simulink model "Concave_hipp"  (R2023a)
settings: Solver=ode3  StartTime=0.0  StopTime=50  FixedStep=0.0001  RelTol=1e-3
values from neighbouring files (symbols this model uses):
  A = A1+A2    [dpdx_linearhipp.m]    (also in main_linear_hipp.m)
  B = [zeros(3,3);diag([1/M1,1/M2,1/M3])]    [dpdx_linearhipp.m]    (also in main_linear_hipp.m)
  Kall = cat(1,Kall,K_)    [main_linear_hipp.m]
  m = 3    [dpdx_linearhipp.m]    (also in main_linear_hipp.m = size(B',1))
  Pall = cat(1,Pall,P_)    [main_linear_hipp.m]
  R0q = Rb    [main_linear_hipp.m]
  rho = zeros(N,1)    [main_linear_hipp.m]
  rhospan = linspace(0,rhom,1000)    [main_linear_hipp.m]
  umax = [0.0288 0.5772 0.5772]    [main_linear_hipp.m]
  x0 = [pi/6;pi/4;pi/3;1;1;1]    [main_linear_hipp.m]
undefined symbols (not defined in the file or in its folder): Kb, Pb, Pcq
settings Model: Creator=fansh  LastModifiedBy=fansh
settings DebuggingCC: MultiTaskCondExecSysMsg=none  MultiTaskRateTransMsg=warning  TasksWithSamePriorityMsg=none  SigSpecEnsureSampleTimeMsg=none  UnknownTsInhSupMsg=none  SFUnexpectedBacktrackingDiag=none

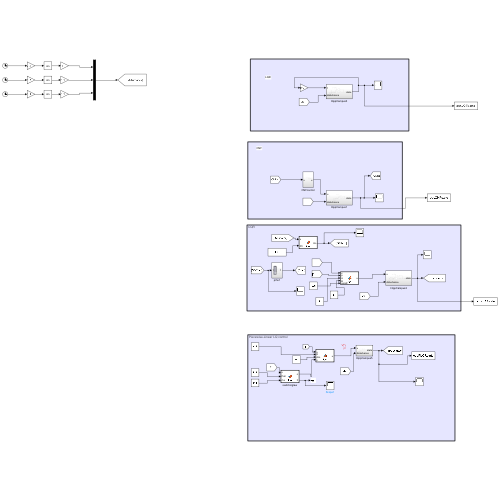
[thumbnail: Simulink's stored preview of the top-level diagram]
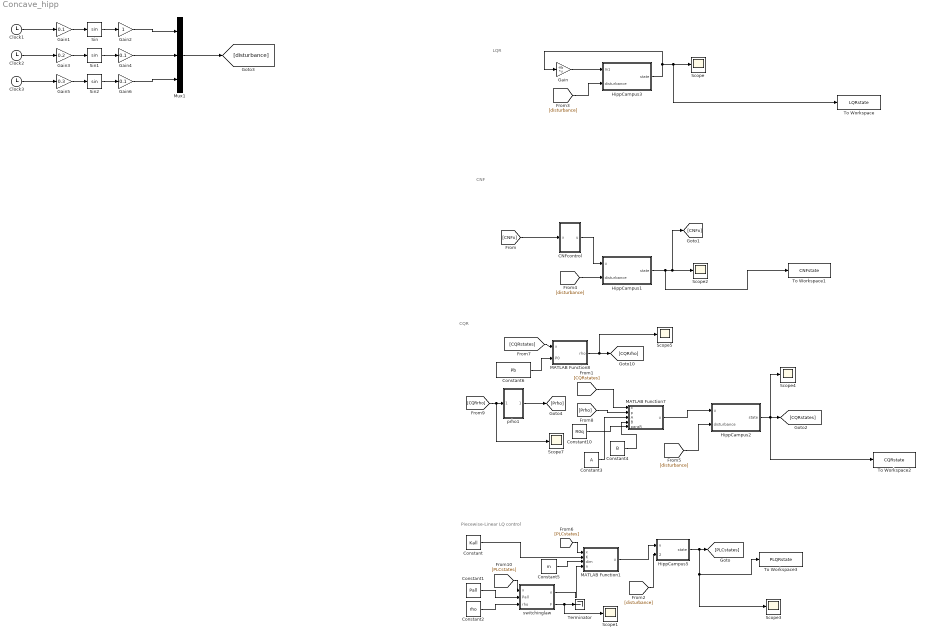
== system Concave_hipp ==
  note: CNF
  note: LQR
  note: CQR
  note: Piecewise-Linear LQ control
  CNFcontrol : Subsystem
  Clock1 : Clock
  Clock2 : Clock
  Clock3 : Clock
  Constant : Constant  Value=Kall
  Constant1 : Constant  Value=Pall
  Constant10 : Constant  Value=R0q
  Constant2 : Constant  Value=rho
  Constant3 : Constant  Value=A
  Constant4 : Constant  Value=B
  Constant5 : Constant  Value=m
  Constant6 : Constant  Value=Pb
  Gain : Gain  Gain=-Kb  Multiplication=Matrix(K*u)
  Gain1 : Gain  Gain=0.1
  Gain2 : Gain
  Gain3 : Gain  Gain=0.2
  Gain4 : Gain  Gain=0.1
  Gain5 : Gain  Gain=0.3
  Gain6 : Gain  Gain=0.1
  HippCampus1 : Subsystem
  HippCampus2 : Subsystem
  HippCampus3 : Subsystem
  HippCampus5 : Subsystem
  MATLAB Function1 : MATLAB Function  TreatAsAtomicUnit=on
  MATLAB Function7 : MATLAB Function  TreatAsAtomicUnit=on
  MATLAB Function8 : MATLAB Function  TreatAsAtomicUnit=on
  Mux1 : Mux  Inputs=3
  Scope{,1..5,7} (7 alike) : Scope
  Sin : Trigonometry
  Sin1 : Trigonometry
  Sin2 : Trigonometry
  Terminator : Terminator
  To Workspace : ToWorkspace  VariableName=LQRstate  SaveFormat=Timeseries  SampleTime=-1
  To Workspace1 : ToWorkspace  VariableName=CNFstate  SaveFormat=Timeseries  SampleTime=-1
  To Workspace2 : ToWorkspace  VariableName=CQRstate  SaveFormat=Timeseries  SampleTime=-1
  To Workspace3 : ToWorkspace  VariableName=PLQRstate  SaveFormat=Timeseries  SampleTime=-1
  prho1 : Subsystem
  switchinglaw : MATLAB Function  TreatAsAtomicUnit=on
  wires:
  HippCampus3/1(state) -> To Workspace/1, Scope/1, Gain/1
  Gain/1 -> HippCampus3/1(In1)
  Clock1/1 -> Gain1/1
  Gain1/1 -> Sin/1
  Sin/1 -> Gain2/1
  Sin1/1 -> Gain4/1
  Clock2/1 -> Gain3/1
  Gain3/1 -> Sin1/1
  Sin2/1 -> Gain6/1
  Clock3/1 -> Gain5/1
  Gain5/1 -> Sin2/1
  Gain2/1 -> Mux1/1
  Gain4/1 -> Mux1/2
  Gain6/1 -> Mux1/3
  Mux1/1 -> [disturbance]
  HippCampus1/1(state) -> To Workspace1/1, Scope2/1, [CNFx]
  [Prho] -> MATLAB Function7/2(p)
  [CQRrho] -> Scope7/1, prho1/1(In1)
  HippCampus2/1(state) -> To Workspace2/1, Scope4/1, [CQRstates]
  prho1/1(Out1) -> [Prho]
  Constant10/1 -> MATLAB Function7/5(paraR)
  MATLAB Function8/1(rho) -> Scope5/1, [CQRrho]
  [CQRstates] -> MATLAB Function8/1(x)
  Constant6/1 -> MATLAB Function8/2(P0)
  MATLAB Function7/1(u) -> HippCampus2/1(u)
  [CQRstates] -> MATLAB Function7/1(x)
  [disturbance] -> HippCampus3/2(disturbance)
  [disturbance] -> HippCampus1/2(disturbance)
  [CNFx] -> CNFcontrol/1(x)
  CNFcontrol/1(u) -> HippCampus1/1(u)
  [disturbance] -> HippCampus2/2(disturbance)
  Constant/1 -> MATLAB Function1/2(K)
  [PLCstates] -> switchinglaw/1(x)
  switchinglaw/2(F) -> Scope1/1, Terminator/1
  switchinglaw/1(n) -> MATLAB Function1/4(n)
  HippCampus5/1(state) -> Scope3/1, To Workspace3/1, [PLCstates]
  ? -> ?
  [PLCstates] -> MATLAB Function1/1(x)
  Constant1/1 -> switchinglaw/2(Pall)
  MATLAB Function1/1(u) -> HippCampus5/1(u)
  Constant2/1 -> switchinglaw/3(rho)
  Constant5/1 -> MATLAB Function1/3(dim)
  [disturbance] -> HippCampus5/2(disturbance)
  Constant3/1 -> MATLAB Function7/3(A)
  Constant4/1 -> MATLAB Function7/4(B)

== system Concave_hipp/CNFcontrol ==
  x : Inport
  Constant : Constant  Value=200
  Constant1 : Constant  Value=Kb
  Constant2 : Constant  Value=Pb
  MATLAB Function1 : MATLAB Function  TreatAsAtomicUnit=on
  MATLAB Function2 : MATLAB Function  TreatAsAtomicUnit=on
  u : Outport
  wires:
  MATLAB Function2/1(rho) -> MATLAB Function1/3(rho)
  MATLAB Function1/1(u) -> u/1
  x/1 -> MATLAB Function2/1(x), MATLAB Function1/1(x)
  Constant/1 -> MATLAB Function1/4(k)
  Constant1/1 -> MATLAB Function1/2(Kb)
  Constant2/1 -> MATLAB Function2/2(Pb)

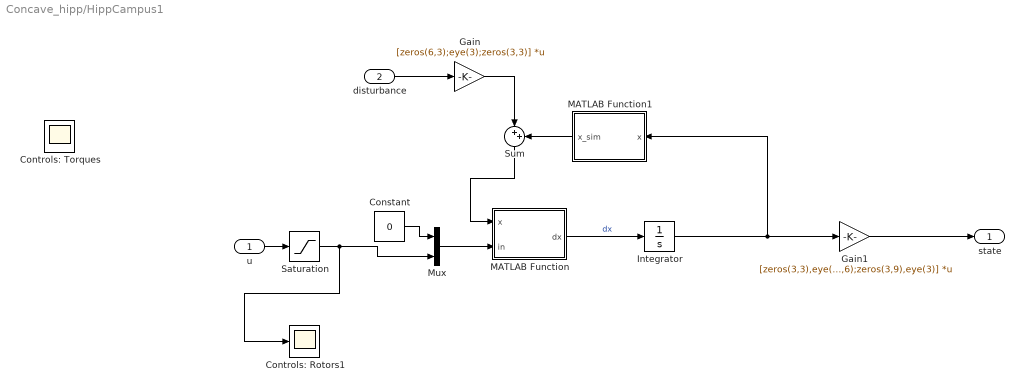
== system Concave_hipp/HippCampus1 ==
  u : Inport
  disturbance : Inport  Port=2
  Constant : Constant  Value=0
  Controls: Rotors1 : Scope
  Controls: Torques : Scope
  Gain : Gain  Gain=[zeros(6,3);eye(3);zeros(3,3)]  Multiplication=Matrix(K*u)
  Gain1 : Gain  Gain=[zeros(3,3),eye(3),zeros(3,6);zeros(3,9),eye(3)]  Multiplication=Matrix(K*u)
  Integrator : Integrator  InitialCondition=[zeros(3,1);x0(1:3);zeros(3,1);x0(4:6)]
  MATLAB Function : MATLAB Function  TreatAsAtomicUnit=on
  MATLAB Function1 : MATLAB Function  TreatAsAtomicUnit=on
  Mux : Mux  Inputs=2
  Saturation : Saturate  UpperLimit=umax'  LowerLimit=-umax'
  Sum : Sum  Inputs=|++
  state : Outport
  wires:
  MATLAB Function/1(dx) -> Integrator/1  "dx"
  Integrator/1 -> Gain1/1, MATLAB Function1/1(x)
  disturbance/1 -> Gain/1
  Gain/1 -> Sum/1
  Sum/1 -> MATLAB Function/1(x)
  MATLAB Function1/1(x_sim) -> Sum/2
  Gain1/1 -> state/1
  Mux/1 -> MATLAB Function/2(in)
  Saturation/1 -> Controls: Rotors1/1, Mux/2
  Constant/1 -> Mux/1
  u/1 -> Saturation/1

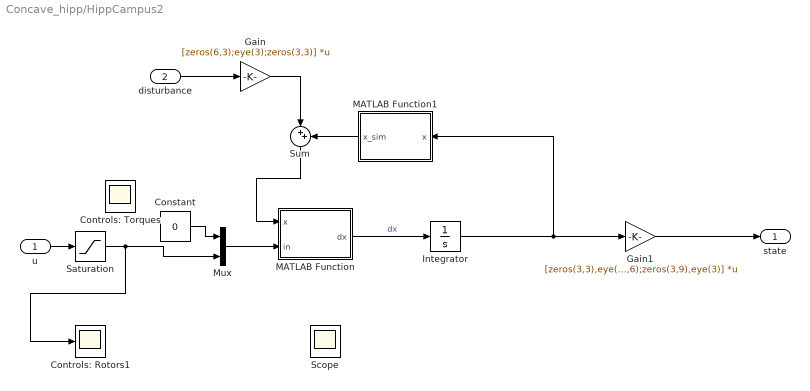
== system Concave_hipp/HippCampus2 ==
  u : Inport
  disturbance : Inport  Port=2
  Constant : Constant  Value=0
  Controls: Rotors1 : Scope
  Controls: Torques : Scope
  Gain : Gain  Gain=[zeros(6,3);eye(3);zeros(3,3)]  Multiplication=Matrix(K*u)
  Gain1 : Gain  Gain=[zeros(3,3),eye(3),zeros(3,6);zeros(3,9),eye(3)]  Multiplication=Matrix(K*u)
  Integrator : Integrator  InitialCondition=[zeros(3,1);x0(1:3);zeros(3,1);x0(4:6)]
  MATLAB Function : MATLAB Function  TreatAsAtomicUnit=on
  MATLAB Function1 : MATLAB Function  TreatAsAtomicUnit=on
  Mux : Mux  Inputs=2
  Saturation : Saturate  UpperLimit=umax'  LowerLimit=-umax'
  Scope : Scope
  Sum : Sum  Inputs=|++
  state : Outport
  wires:
  MATLAB Function/1(dx) -> Integrator/1  "dx"
  Integrator/1 -> Gain1/1, MATLAB Function1/1(x)
  disturbance/1 -> Gain/1
  Gain/1 -> Sum/1
  Sum/1 -> MATLAB Function/1(x)
  MATLAB Function1/1(x_sim) -> Sum/2
  Gain1/1 -> state/1
  Mux/1 -> MATLAB Function/2(in)
  Saturation/1 -> Controls: Rotors1/1, Mux/2
  Constant/1 -> Mux/1
  u/1 -> Saturation/1
  ? -> Scope/1

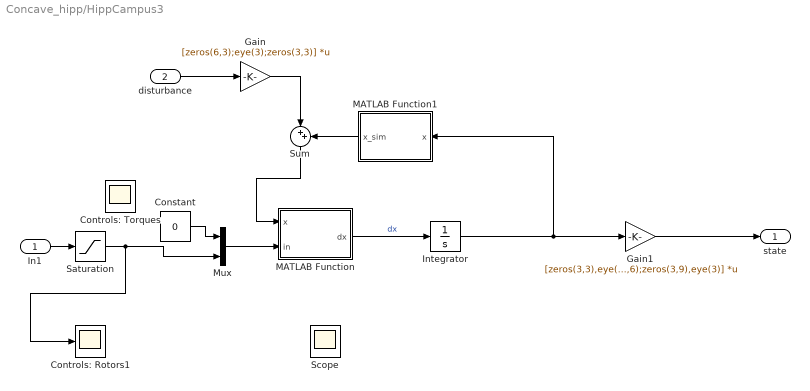
== system Concave_hipp/HippCampus3 ==
  In1 : Inport
  disturbance : Inport  Port=2
  Constant : Constant  Value=0
  Controls: Rotors1 : Scope
  Controls: Torques : Scope
  Gain : Gain  Gain=[zeros(6,3);eye(3);zeros(3,3)]  Multiplication=Matrix(K*u)
  Gain1 : Gain  Gain=[zeros(3,3),eye(3),zeros(3,6);zeros(3,9),eye(3)]  Multiplication=Matrix(K*u)
  Integrator : Integrator  InitialCondition=[zeros(3,1);x0(1:3);zeros(3,1);x0(4:6)]
  MATLAB Function : MATLAB Function  TreatAsAtomicUnit=on
  MATLAB Function1 : MATLAB Function  TreatAsAtomicUnit=on
  Mux : Mux  Inputs=2
  Saturation : Saturate  UpperLimit=umax'  LowerLimit=-umax'
  Scope : Scope
  Sum : Sum  Inputs=|++
  state : Outport
  wires:
  MATLAB Function/1(dx) -> Integrator/1  "dx"
  Integrator/1 -> Gain1/1, MATLAB Function1/1(x)
  disturbance/1 -> Gain/1
  Gain/1 -> Sum/1
  Sum/1 -> MATLAB Function/1(x)
  MATLAB Function1/1(x_sim) -> Sum/2
  Gain1/1 -> state/1
  Mux/1 -> MATLAB Function/2(in)
  Saturation/1 -> Controls: Rotors1/1, Mux/2
  Constant/1 -> Mux/1
  In1/1 -> Saturation/1
  ? -> Scope/1

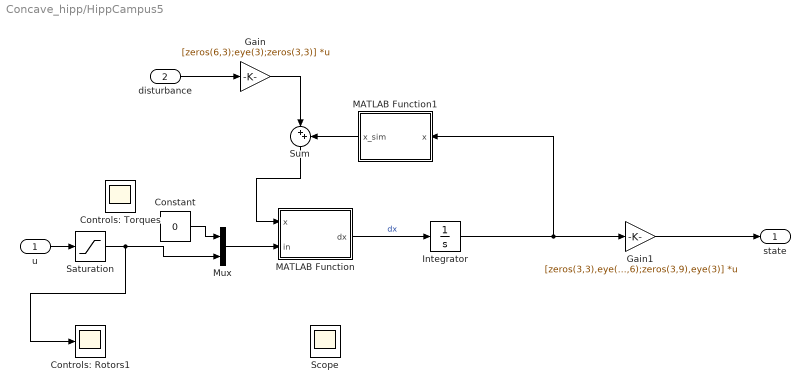
== system Concave_hipp/HippCampus5 ==
  u : Inport
  disturbance : Inport  Port=2
  Constant : Constant  Value=0
  Controls: Rotors1 : Scope
  Controls: Torques : Scope
  Gain : Gain  Gain=[zeros(6,3);eye(3);zeros(3,3)]  Multiplication=Matrix(K*u)
  Gain1 : Gain  Gain=[zeros(3,3),eye(3),zeros(3,6);zeros(3,9),eye(3)]  Multiplication=Matrix(K*u)
  Integrator : Integrator  InitialCondition=[zeros(3,1);x0(1:3);zeros(3,1);x0(4:6)]
  MATLAB Function : MATLAB Function  TreatAsAtomicUnit=on
  MATLAB Function1 : MATLAB Function  TreatAsAtomicUnit=on
  Mux : Mux  Inputs=2
  Saturation : Saturate  UpperLimit=umax'  LowerLimit=-umax'
  Scope : Scope
  Sum : Sum  Inputs=|++
  state : Outport
  wires:
  MATLAB Function/1(dx) -> Integrator/1  "dx"
  Integrator/1 -> Gain1/1, MATLAB Function1/1(x)
  disturbance/1 -> Gain/1
  Gain/1 -> Sum/1
  Sum/1 -> MATLAB Function/1(x)
  MATLAB Function1/1(x_sim) -> Sum/2
  Gain1/1 -> state/1
  Mux/1 -> MATLAB Function/2(in)
  Saturation/1 -> Controls: Rotors1/1, Mux/2
  Constant/1 -> Mux/1
  u/1 -> Saturation/1
  ? -> Scope/1

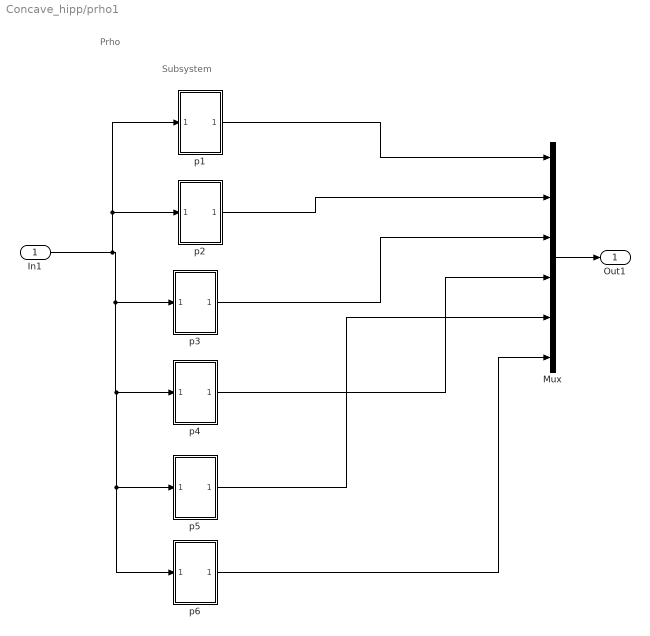
== system Concave_hipp/prho1 ==
  note: Prho
  note: Subsystem
  In1 : Inport
  Mux : Mux  Inputs=6
  p1 : Subsystem
  p2 : Subsystem
  p3 : Subsystem
  p4 : Subsystem
  p5 : Subsystem
  p6 : Subsystem
  Out1 : Outport
  wires:
  p4/1(Out1) -> Mux/4
  In1/1 -> p6/1(In1), p5/1(In1), p4/1(In1), p3/1(In1), p2/1(In1), p1/1(In1)
  Mux/1 -> Out1/1
  p1/1(Out1) -> Mux/1
  p3/1(Out1) -> Mux/3
  p2/1(Out1) -> Mux/2
  p5/1(Out1) -> Mux/5
  p6/1(Out1) -> Mux/6

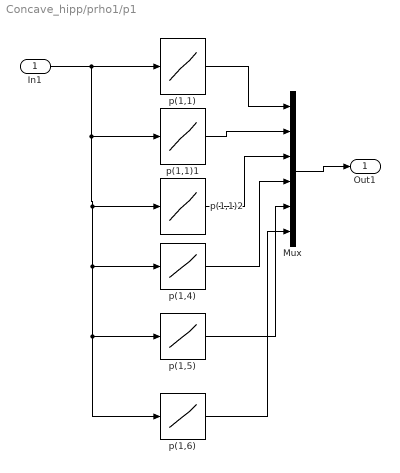
== system Concave_hipp/prho1/p1 ==
  In1 : Inport
  Mux : Mux  Inputs=6
  p(1,1) : Lookup_n-D  NumberOfTableDimensions=1  BreakpointsForDimension1=rhospan  Table=Pcq(:,1)  InterpMethod=Linear Lagrange  InternalRulePriority=Speed  RndMeth=Simplest
  p(1,1)1 : Lookup_n-D  NumberOfTableDimensions=1  BreakpointsForDimension1=rhospan  Table=Pcq(:,2)  InterpMethod=Linear Lagrange  InternalRulePriority=Speed  RndMeth=Simplest
  p(1,1)2 : Lookup_n-D  NumberOfTableDimensions=1  BreakpointsForDimension1=rhospan  Table=Pcq(:,3)  InterpMethod=Linear Lagrange  InternalRulePriority=Speed  RndMeth=Simplest
  p(1,4) : Lookup_n-D  NumberOfTableDimensions=1  BreakpointsForDimension1=rhospan  Table=Pcq(:,4)  InterpMethod=Linear Lagrange  InternalRulePriority=Speed  RndMeth=Simplest
  p(1,5) : Lookup_n-D  NumberOfTableDimensions=1  BreakpointsForDimension1=rhospan  Table=Pcq(:,5)  InterpMethod=Linear Lagrange  InternalRulePriority=Speed  RndMeth=Simplest
  p(1,6) : Lookup_n-D  NumberOfTableDimensions=1  BreakpointsForDimension1=rhospan  Table=Pcq(:,6)  InterpMethod=Linear Lagrange  InternalRulePriority=Speed  RndMeth=Simplest
  Out1 : Outport
  wires:
  p(1,1)1/1 -> Mux/2
  p(1,4)/1 -> Mux/4
  In1/1 -> p(1,1)1/1, p(1,1)2/1, p(1,6)/1, p(1,5)/1, p(1,4)/1, p(1,1)/1
  p(1,1)/1 -> Mux/1
  p(1,1)2/1 -> Mux/3
  Mux/1 -> Out1/1
  p(1,5)/1 -> Mux/5
  p(1,6)/1 -> Mux/6

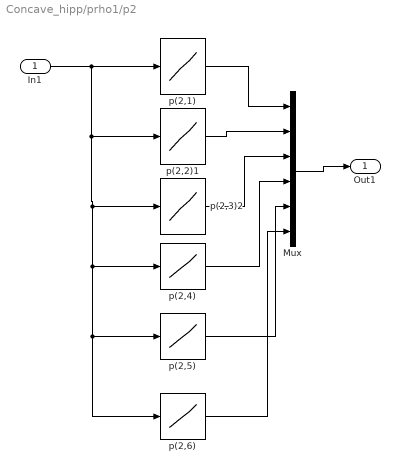
== system Concave_hipp/prho1/p2 ==
  In1 : Inport
  Mux : Mux  Inputs=6
  p(2,1) : Lookup_n-D  NumberOfTableDimensions=1  BreakpointsForDimension1=rhospan  Table=Pcq(:,7)  InterpMethod=Linear Lagrange  InternalRulePriority=Speed  RndMeth=Simplest
  p(2,2)1 : Lookup_n-D  NumberOfTableDimensions=1  BreakpointsForDimension1=rhospan  Table=Pcq(:,8)  InterpMethod=Linear Lagrange  InternalRulePriority=Speed  RndMeth=Simplest
  p(2,3)2 : Lookup_n-D  NumberOfTableDimensions=1  BreakpointsForDimension1=rhospan  Table=Pcq(:,9)  InterpMethod=Linear Lagrange  InternalRulePriority=Speed  RndMeth=Simplest
  p(2,4) : Lookup_n-D  NumberOfTableDimensions=1  BreakpointsForDimension1=rhospan  Table=Pcq(:,10)  InterpMethod=Linear Lagrange  InternalRulePriority=Speed  RndMeth=Simplest
  p(2,5) : Lookup_n-D  NumberOfTableDimensions=1  BreakpointsForDimension1=rhospan  Table=Pcq(:,11)  InterpMethod=Linear Lagrange  InternalRulePriority=Speed  RndMeth=Simplest
  p(2,6) : Lookup_n-D  NumberOfTableDimensions=1  BreakpointsForDimension1=rhospan  Table=Pcq(:,12)  InterpMethod=Linear Lagrange  InternalRulePriority=Speed  RndMeth=Simplest
  Out1 : Outport
  wires:
  p(2,2)1/1 -> Mux/2
  p(2,4)/1 -> Mux/4
  In1/1 -> p(2,2)1/1, p(2,3)2/1, p(2,6)/1, p(2,5)/1, p(2,4)/1, p(2,1)/1
  p(2,1)/1 -> Mux/1
  p(2,3)2/1 -> Mux/3
  Mux/1 -> Out1/1
  p(2,5)/1 -> Mux/5
  p(2,6)/1 -> Mux/6

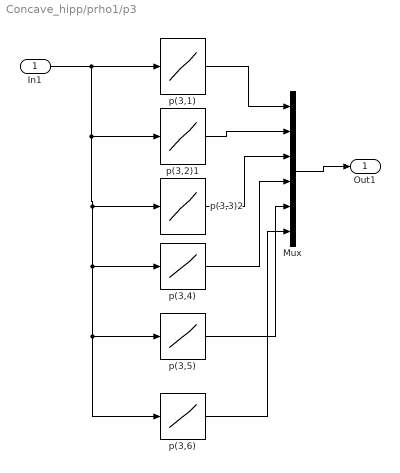
== system Concave_hipp/prho1/p3 ==
  In1 : Inport
  Mux : Mux  Inputs=6
  p(3,1) : Lookup_n-D  NumberOfTableDimensions=1  BreakpointsForDimension1=rhospan  Table=Pcq(:,13)  InterpMethod=Linear Lagrange  InternalRulePriority=Speed  RndMeth=Simplest
  p(3,2)1 : Lookup_n-D  NumberOfTableDimensions=1  BreakpointsForDimension1=rhospan  Table=Pcq(:,14)  InterpMethod=Linear Lagrange  InternalRulePriority=Speed  RndMeth=Simplest
  p(3,3)2 : Lookup_n-D  NumberOfTableDimensions=1  BreakpointsForDimension1=rhospan  Table=Pcq(:,15)  InterpMethod=Linear Lagrange  InternalRulePriority=Speed  RndMeth=Simplest
  p(3,4) : Lookup_n-D  NumberOfTableDimensions=1  BreakpointsForDimension1=rhospan  Table=Pcq(:,16)  InterpMethod=Linear Lagrange  InternalRulePriority=Speed  RndMeth=Simplest
  p(3,5) : Lookup_n-D  NumberOfTableDimensions=1  BreakpointsForDimension1=rhospan  Table=Pcq(:,17)  InterpMethod=Linear Lagrange  InternalRulePriority=Speed  RndMeth=Simplest
  p(3,6) : Lookup_n-D  NumberOfTableDimensions=1  BreakpointsForDimension1=rhospan  Table=Pcq(:,18)  InterpMethod=Linear Lagrange  InternalRulePriority=Speed  RndMeth=Simplest
  Out1 : Outport
  wires:
  p(3,2)1/1 -> Mux/2
  p(3,4)/1 -> Mux/4
  In1/1 -> p(3,2)1/1, p(3,3)2/1, p(3,6)/1, p(3,5)/1, p(3,4)/1, p(3,1)/1
  p(3,1)/1 -> Mux/1
  p(3,3)2/1 -> Mux/3
  Mux/1 -> Out1/1
  p(3,5)/1 -> Mux/5
  p(3,6)/1 -> Mux/6

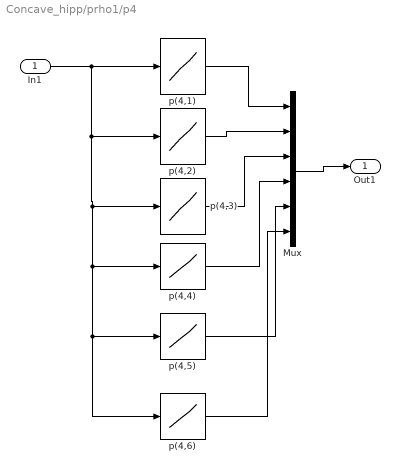
== system Concave_hipp/prho1/p4 ==
  In1 : Inport
  Mux : Mux  Inputs=6
  p(4,1) : Lookup_n-D  NumberOfTableDimensions=1  BreakpointsForDimension1=rhospan  Table=Pcq(:,19)  InterpMethod=Linear Lagrange  InternalRulePriority=Speed  RndMeth=Simplest
  p(4,2) : Lookup_n-D  NumberOfTableDimensions=1  BreakpointsForDimension1=rhospan  Table=Pcq(:,20)  InterpMethod=Linear Lagrange  InternalRulePriority=Speed  RndMeth=Simplest
  p(4,3) : Lookup_n-D  NumberOfTableDimensions=1  BreakpointsForDimension1=rhospan  Table=Pcq(:,21)  InterpMethod=Linear Lagrange  InternalRulePriority=Speed  RndMeth=Simplest
  p(4,4) : Lookup_n-D  NumberOfTableDimensions=1  BreakpointsForDimension1=rhospan  Table=Pcq(:,22)  InterpMethod=Linear Lagrange  InternalRulePriority=Speed  RndMeth=Simplest
  p(4,5) : Lookup_n-D  NumberOfTableDimensions=1  BreakpointsForDimension1=rhospan  Table=Pcq(:,23)  InterpMethod=Linear Lagrange  InternalRulePriority=Speed  RndMeth=Simplest
  p(4,6) : Lookup_n-D  NumberOfTableDimensions=1  BreakpointsForDimension1=rhospan  Table=Pcq(:,24)  InterpMethod=Linear Lagrange  InternalRulePriority=Speed  RndMeth=Simplest
  Out1 : Outport
  wires:
  p(4,2)/1 -> Mux/2
  p(4,4)/1 -> Mux/4
  In1/1 -> p(4,2)/1, p(4,3)/1, p(4,6)/1, p(4,5)/1, p(4,4)/1, p(4,1)/1
  p(4,1)/1 -> Mux/1
  p(4,3)/1 -> Mux/3
  Mux/1 -> Out1/1
  p(4,5)/1 -> Mux/5
  p(4,6)/1 -> Mux/6

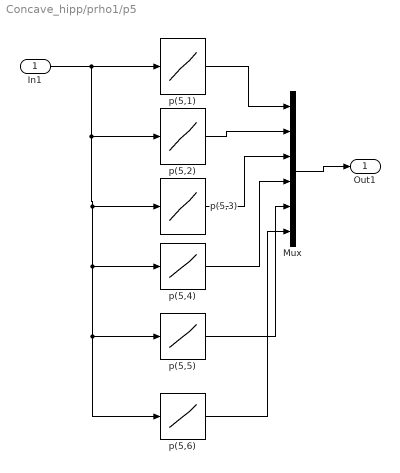
== system Concave_hipp/prho1/p5 ==
  In1 : Inport
  Mux : Mux  Inputs=6
  p(5,1) : Lookup_n-D  NumberOfTableDimensions=1  BreakpointsForDimension1=rhospan  Table=Pcq(:,25)  InterpMethod=Linear Lagrange  InternalRulePriority=Speed  RndMeth=Simplest
  p(5,2) : Lookup_n-D  NumberOfTableDimensions=1  BreakpointsForDimension1=rhospan  Table=Pcq(:,26)  InterpMethod=Linear Lagrange  InternalRulePriority=Speed  RndMeth=Simplest
  p(5,3) : Lookup_n-D  NumberOfTableDimensions=1  BreakpointsForDimension1=rhospan  Table=Pcq(:,27)  InterpMethod=Linear Lagrange  InternalRulePriority=Speed  RndMeth=Simplest
  p(5,4) : Lookup_n-D  NumberOfTableDimensions=1  BreakpointsForDimension1=rhospan  Table=Pcq(:,28)  InterpMethod=Linear Lagrange  InternalRulePriority=Speed  RndMeth=Simplest
  p(5,5) : Lookup_n-D  NumberOfTableDimensions=1  BreakpointsForDimension1=rhospan  Table=Pcq(:,29)  InterpMethod=Linear Lagrange  InternalRulePriority=Speed  RndMeth=Simplest
  p(5,6) : Lookup_n-D  NumberOfTableDimensions=1  BreakpointsForDimension1=rhospan  Table=Pcq(:,30)  InterpMethod=Linear Lagrange  InternalRulePriority=Speed  RndMeth=Simplest
  Out1 : Outport
  wires:
  p(5,2)/1 -> Mux/2
  p(5,4)/1 -> Mux/4
  In1/1 -> p(5,2)/1, p(5,3)/1, p(5,6)/1, p(5,5)/1, p(5,4)/1, p(5,1)/1
  p(5,1)/1 -> Mux/1
  p(5,3)/1 -> Mux/3
  Mux/1 -> Out1/1
  p(5,5)/1 -> Mux/5
  p(5,6)/1 -> Mux/6

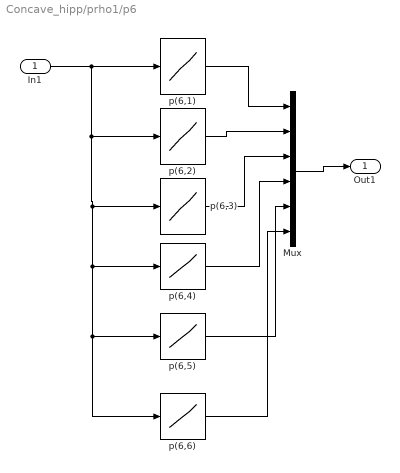
== system Concave_hipp/prho1/p6 ==
  In1 : Inport
  Mux : Mux  Inputs=6
  p(6,1) : Lookup_n-D  NumberOfTableDimensions=1  BreakpointsForDimension1=rhospan  Table=Pcq(:,31)  InterpMethod=Linear Lagrange  InternalRulePriority=Speed  RndMeth=Simplest
  p(6,2) : Lookup_n-D  NumberOfTableDimensions=1  BreakpointsForDimension1=rhospan  Table=Pcq(:,32)  InterpMethod=Linear Lagrange  InternalRulePriority=Speed  RndMeth=Simplest
  p(6,3) : Lookup_n-D  NumberOfTableDimensions=1  BreakpointsForDimension1=rhospan  Table=Pcq(:,33)  InterpMethod=Linear Lagrange  InternalRulePriority=Speed  RndMeth=Simplest
  p(6,4) : Lookup_n-D  NumberOfTableDimensions=1  BreakpointsForDimension1=rhospan  Table=Pcq(:,34)  InterpMethod=Linear Lagrange  InternalRulePriority=Speed  RndMeth=Simplest
  p(6,5) : Lookup_n-D  NumberOfTableDimensions=1  BreakpointsForDimension1=rhospan  Table=Pcq(:,35)  InterpMethod=Linear Lagrange  InternalRulePriority=Speed  RndMeth=Simplest
  p(6,6) : Lookup_n-D  NumberOfTableDimensions=1  BreakpointsForDimension1=rhospan  Table=Pcq(:,36)  InterpMethod=Linear Lagrange  InternalRulePriority=Speed  RndMeth=Simplest
  Out1 : Outport
  wires:
  p(6,2)/1 -> Mux/2
  p(6,4)/1 -> Mux/4
  In1/1 -> p(6,2)/1, p(6,3)/1, p(6,6)/1, p(6,5)/1, p(6,4)/1, p(6,1)/1
  p(6,1)/1 -> Mux/1
  p(6,3)/1 -> Mux/3
  Mux/1 -> Out1/1
  p(6,5)/1 -> Mux/5
  p(6,6)/1 -> Mux/6

== matlab function Concave_hipp/HippCampus5/MATLAB Function1 ==
  data: x input; x_sim output
function x_sim = fcn(x)
x(1:3) = zeros(3,1);
x(7:9) = zeros(3,1);
x_sim = x;
end

== matlab function Concave_hipp/HippCampus3/MATLAB Function1 ==
  data: x input; x_sim output
function x_sim = fcn(x)
x(1:3) = zeros(3,1);
x(7:9) = zeros(3,1);
x_sim = x;
end

== matlab function Concave_hipp/HippCampus1/MATLAB Function ==
  data: x input; dx output; in input

function dx = fcn(x, in)
zg    =  0.05;    % [m]
g     =  9.81;    % [m/s^2]

m     =  1.43;    % [kg]
Ix    = 0.00241; % [kgm^2]
Iy    = 0.01072; % [kgm^2]
Iz    = 0.01072; % [kgm^2]
Xudot = -1.11;    % [kg]
Yvdot = -2.80;    % [kg]
Zwdot = -2.80;    % [kg]
Kpdot = -0.0018;  % [kgm^2]
Mqdot = -0.0095;  % [kgm^2]
Nrdot = -0.0095;  % [kgm^2]
Xu    = -4.56;    % [kg/m]
Yv    = -17.36;   % [kg/m]
Zw    = -17.36;   % [kg/m]
Kp    = -0.0028;  % [kgm^2]
Mq    = -0.0476;  % [kgm^2]
Nr    = -0.0476;  % [kgm^2]
% Extract states into more readable form
phi = x( 4); theta = x( 5);
u   = x( 7); v     = x( 8); w   = x( 9);
p   = x(10); q     = x(11); r   = x(12);
nu  = x(7:12);

% Construct rotational tensor
R = body_frame_rotation(x(4:6));

% Construct velocity transformation tensor
T = [ 1  sin(phi)*tan(theta)   cos(phi)*tan(theta) ;
    0  cos(phi)             -sin(phi)            ;
    0  sin(phi)/cos(theta)   cos(phi)/cos(theta) ];
J = [ R         zeros(3) ;
    zeros(3)  T        ];

% Calculate mass matrix
Ma  = -diag([Xudot, Yvdot, Zwdot, Kpdot, Mqdot, Nrdot]);
Mrb =  diag([m,  m,  m, Ix, Iy, Iz]);
M = Ma + Mrb;

% Compute hydrostatic load
gravity = zg * g * m;
G = [ 0; 0; 0; gravity * cos(theta) * sin(phi); gravity * sin(theta); 0 ];

% Construct coriolis matrix, see Fossen 2011, Theorem 3.2
C12 = -skew(M(1:3,1:3) * nu(1:3));
C = [ zeros(3)   C12                        ;
    C12       -skew(M(4:6,4:6) * nu(4:6)) ];

% Construct damping matrix
D = -diag([Xu * abs(u), Yv * abs(v),...
    Zw * abs(w), Kp * abs(p),...
    Mq * abs(q), Nr * abs(r)]);

% Build state space equations
tau  = [ in(1); 0; 0; in(2:4) ];

dx       = zeros(12,1);
dx(1:6)  = J*nu;
dx(7:12) = M \ (tau - (C+D)*nu - G);
end

== matlab function Concave_hipp/HippCampus3/MATLAB Function ==
  data: x input; dx output; in input

function dx = fcn(x, in)
zg    =  0.05;    % [m]
g     =  9.81;    % [m/s^2]

m     =  1.43;    % [kg]
Ix    = 0.00241; % [kgm^2]
Iy    = 0.01072; % [kgm^2]
Iz    = 0.01072; % [kgm^2]
Xudot = -1.11;    % [kg]
Yvdot = -2.80;    % [kg]
Zwdot = -2.80;    % [kg]
Kpdot = -0.0018;  % [kgm^2]
Mqdot = -0.0095;  % [kgm^2]
Nrdot = -0.0095;  % [kgm^2]
Xu    = -4.56;    % [kg/m]
Yv    = -17.36;   % [kg/m]
Zw    = -17.36;   % [kg/m]
Kp    = -0.0028;  % [kgm^2]
Mq    = -0.0476;  % [kgm^2]
Nr    = -0.0476;  % [kgm^2]
% Extract states into more readable form
phi = x( 4); theta = x( 5);
u   = x( 7); v     = x( 8); w   = x( 9);
p   = x(10); q     = x(11); r   = x(12);
nu  = x(7:12);

% Construct rotational tensor
R = body_frame_rotation(x(4:6));

% Construct velocity transformation tensor
T = [ 1  sin(phi)*tan(theta)   cos(phi)*tan(theta) ;
    0  cos(phi)             -sin(phi)            ;
    0  sin(phi)/cos(theta)   cos(phi)/cos(theta) ];
J = [ R         zeros(3) ;
    zeros(3)  T        ];

% Calculate mass matrix
Ma  = -diag([Xudot, Yvdot, Zwdot, Kpdot, Mqdot, Nrdot]);
Mrb =  diag([m,  m,  m, Ix, Iy, Iz]);
M = Ma + Mrb;

% Compute hydrostatic load
gravity = zg * g * m;
G = [ 0; 0; 0; gravity * cos(theta) * sin(phi); gravity * sin(theta); 0 ];

% Construct coriolis matrix, see Fossen 2011, Theorem 3.2
C12 = -skew(M(1:3,1:3) * nu(1:3));
C = [ zeros(3)   C12                        ;
    C12       -skew(M(4:6,4:6) * nu(4:6)) ];

% Construct damping matrix
D = -diag([Xu * abs(u), Yv * abs(v),...
    Zw * abs(w), Kp * abs(p),...
    Mq * abs(q), Nr * abs(r)]);

% Build state space equations
tau  = [ in(1); 0; 0; in(2:4) ];

dx       = zeros(12,1);
dx(1:6)  = J*nu;
dx(7:12) = M \ (tau - (C+D)*nu - G);
end

== matlab function Concave_hipp/HippCampus1/MATLAB Function1 ==
  data: x input; x_sim output
function x_sim = fcn(x)
x(1:3) = zeros(3,1);
x(7:9) = zeros(3,1);
x_sim = x;
end

== matlab function Concave_hipp/CNFcontrol/MATLAB Function1 ==
  data: x input; u output; Kb input; rho input; k input
function u= fcn(x,Kb,rho,k)
u = - (1+k*exp(-0.65*(rho)))*Kb*x;

== matlab function Concave_hipp/CNFcontrol/MATLAB Function2 ==
  data: x input; rho output; Pb input
function rho = fcn(x,Pb)

rho = x'*Pb*x;

== matlab function Concave_hipp/HippCampus2/MATLAB Function ==
  data: x input; dx output; in input

function dx = fcn(x, in)
zg    =  0.05;    % [m]
g     =  9.81;    % [m/s^2]

m     =  1.43;    % [kg]
Ix    = 0.00241; % [kgm^2]
Iy    = 0.01072; % [kgm^2]
Iz    = 0.01072; % [kgm^2]
Xudot = -1.11;    % [kg]
Yvdot = -2.80;    % [kg]
Zwdot = -2.80;    % [kg]
Kpdot = -0.0018;  % [kgm^2]
Mqdot = -0.0095;  % [kgm^2]
Nrdot = -0.0095;  % [kgm^2]
Xu    = -4.56;    % [kg/m]
Yv    = -17.36;   % [kg/m]
Zw    = -17.36;   % [kg/m]
Kp    = -0.0028;  % [kgm^2]
Mq    = -0.0476;  % [kgm^2]
Nr    = -0.0476;  % [kgm^2]
% Extract states into more readable form
phi = x( 4); theta = x( 5);
u   = x( 7); v     = x( 8); w   = x( 9);
p   = x(10); q     = x(11); r   = x(12);
nu  = x(7:12);

% Construct rotational tensor
R = body_frame_rotation(x(4:6));

% Construct velocity transformation tensor
T = [ 1  sin(phi)*tan(theta)   cos(phi)*tan(theta) ;
    0  cos(phi)             -sin(phi)            ;
    0  sin(phi)/cos(theta)   cos(phi)/cos(theta) ];
J = [ R         zeros(3) ;
    zeros(3)  T        ];

% Calculate mass matrix
Ma  = -diag([Xudot, Yvdot, Zwdot, Kpdot, Mqdot, Nrdot]);
Mrb =  diag([m,  m,  m, Ix, Iy, Iz]);
M = Ma + Mrb;

% Compute hydrostatic load
gravity = zg * g * m;
G = [ 0; 0; 0; gravity * cos(theta) * sin(phi); gravity * sin(theta); 0 ];

% Construct coriolis matrix, see Fossen 2011, Theorem 3.2
C12 = -skew(M(1:3,1:3) * nu(1:3));
C = [ zeros(3)   C12                        ;
    C12       -skew(M(4:6,4:6) * nu(4:6)) ];

% Construct damping matrix
D = -diag([Xu * abs(u), Yv * abs(v),...
    Zw * abs(w), Kp * abs(p),...
    Mq * abs(q), Nr * abs(r)]);

% Build state space equations
tau  = [ in(1); 0; 0; in(2:4) ];

dx       = zeros(12,1);
dx(1:6)  = J*nu;
dx(7:12) = M \ (tau - (C+D)*nu - G);
end

== matlab function Concave_hipp/HippCampus2/MATLAB Function1 ==
  data: x input; x_sim output
function x_sim = fcn(x)
x(1:3) = zeros(3,1);
x(7:9) = zeros(3,1);
x_sim = x;
end

== matlab function Concave_hipp/MATLAB Function1 ==
  data: x input; u output; K input; dim input; n input
function u = fcn(x,K,dim,n)
udim = dim;
%selector = n*dim-2;
%Kuse = zeros(dim,6);
%Kuse(1,:)=K(n*dim-2,:);
%Kuse(2,:)=K(n*dim-1,:);
%Kuse(3,:)=K(n*dim,:);
%Kuse = K(selector:n*dim,1:6);
%u = zeros(3,1);
%u(1) = -Kuse(1,:)*x;
%u(2) = -Kuse(2,:)*x;
%u(3) = -Kuse(3,:)*x;
d = -K((n*udim-udim+1):(n*udim),:)*x;
u = zeros(3,1);
u(1)=d(1);
u(2)=d(2);
u(3)=d(3);
end

== matlab function Concave_hipp/switchinglaw ==
  data: x input; n output; Pall input; rho input; F output
function [n,F] = fcn(x,Pall,rho)
N = size(rho,1);
i = 1;
xdim = size(Pall',1);
%udim = dim;
F = zeros(N,1);
for i = 1:N
    P = Pall(i*xdim-xdim+1:i*xdim,:);
    F(i) = sign(rho(i)-x'*P*x);
end
n=1;
for i = 1:N-1
    d = F(i)*F(i+1);
    if d<0
        n = i;
    end
end

if F(1)*F(N)>0&&F(1)>0
    n = N;
end
if F(1)*F(N)>0&&F(1)<0
    n = 1;
end

== matlab function Concave_hipp/MATLAB Function7 ==
  data: x input; u output; p input; A input; B input; paraR input
function u= fcn(x,p,A,B,paraR)
R =paraR;

% system matrix

p_ = reshape(p,[6,6]);
P = p_';
R_inv = inv(R);
u = -R_inv*B'*P*x;

== matlab function Concave_hipp/MATLAB Function8 ==
  data: x input; rho output; P0 input
function rho = fcn(x,P0)

rho = x'*P0*x;

== matlab function Concave_hipp/HippCampus5/MATLAB Function ==
  data: x input; dx output; in input

function dx = fcn(x, in)
zg    =  0.05;    % [m]
g     =  9.81;    % [m/s^2]

m     =  1.43;    % [kg]
Ix    = 0.00241; % [kgm^2]
Iy    = 0.01072; % [kgm^2]
Iz    = 0.01072; % [kgm^2]
Xudot = -1.11;    % [kg]
Yvdot = -2.80;    % [kg]
Zwdot = -2.80;    % [kg]
Kpdot = -0.0018;  % [kgm^2]
Mqdot = -0.0095;  % [kgm^2]
Nrdot = -0.0095;  % [kgm^2]
Xu    = -4.56;    % [kg/m]
Yv    = -17.36;   % [kg/m]
Zw    = -17.36;   % [kg/m]
Kp    = -0.0028;  % [kgm^2]
Mq    = -0.0476;  % [kgm^2]
Nr    = -0.0476;  % [kgm^2]
% Extract states into more readable form
phi = x( 4); theta = x( 5);
u   = x( 7); v     = x( 8); w   = x( 9);
p   = x(10); q     = x(11); r   = x(12);
nu  = x(7:12);

% Construct rotational tensor
R = body_frame_rotation(x(4:6));

% Construct velocity transformation tensor
T = [ 1  sin(phi)*tan(theta)   cos(phi)*tan(theta) ;
    0  cos(phi)             -sin(phi)            ;
    0  sin(phi)/cos(theta)   cos(phi)/cos(theta) ];
J = [ R         zeros(3) ;
    zeros(3)  T        ];

% Calculate mass matrix
Ma  = -diag([Xudot, Yvdot, Zwdot, Kpdot, Mqdot, Nrdot]);
Mrb =  diag([m,  m,  m, Ix, Iy, Iz]);
M = Ma + Mrb;

% Compute hydrostatic load
gravity = zg * g * m;
G = [ 0; 0; 0; gravity * cos(theta) * sin(phi); gravity * sin(theta); 0 ];

% Construct coriolis matrix, see Fossen 2011, Theorem 3.2
C12 = -skew(M(1:3,1:3) * nu(1:3));
C = [ zeros(3)   C12                        ;
    C12       -skew(M(4:6,4:6) * nu(4:6)) ];

% Construct damping matrix
D = -diag([Xu * abs(u), Yv * abs(v),...
    Zw * abs(w), Kp * abs(p),...
    Mq * abs(q), Nr * abs(r)]);

% Build state space equations
tau  = [ in(1); 0; 0; in(2:4) ];

dx       = zeros(12,1);
dx(1:6)  = J*nu;
dx(7:12) = M \ (tau - (C+D)*nu - G);
end
